simulink model "RoboCup_ARM"  (R2025b)
settings: Solver=FixedStepAuto  StartTime=0.0  StopTime=inf  FixedStep=0.01  RelTol=1e-3
StartFcn:
  | clear attachToRobot
  | clear attachToTool
undefined symbols (not defined in the file or in its folder): gray, q_grip1, Sim3dSensor
libraries: sim3dlib x5, robotsim3dlib x1, robotcorelib x1, robotmaniplib x1, sim3dcameralib x1
settings Model: SimulationMode=accelerator  Creator=Abhishek  LastModifiedBy=FYF
settings DataIOCC: SaveOutput=off  SignalLogging=off  SaveTime=off

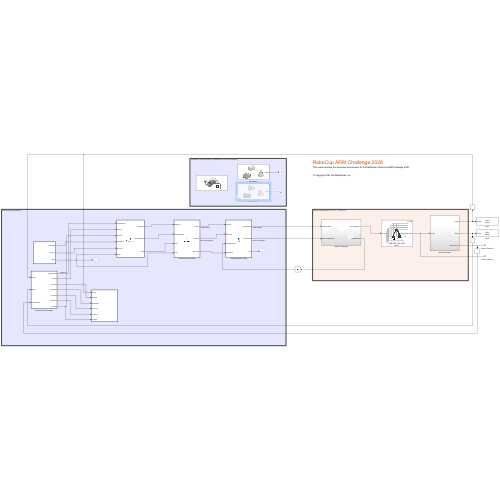
[thumbnail: Simulink's stored preview of the top-level diagram]
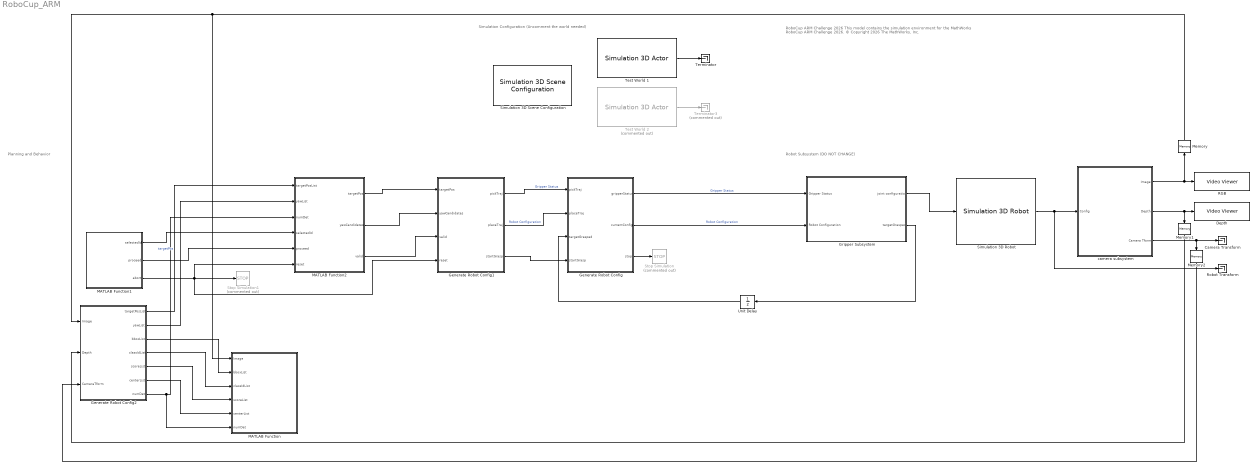
== system RoboCup_ARM ==
  note: Robot Subsystem (DO NOT CHANGE)
  note: Planning and Behavior
  note: Simulation Configuration (Uncomment the world needed)
  note: RoboCup ARM Challenge 2026
      | This model contains the simulation environment for the MathWorks RoboCup ARM Challenge 2026.
      |
      | © Copyright 2026 The MathWorks, Inc.
  Camera Transform : Terminator
  Depth : VideoViewer  colormapValue=gray(256)  FigPos=[1244 879.666666666667 418 304]
  Generate Robot Config : MATLAB Function  TreatAsAtomicUnit=on
  Generate Robot Config1 : MATLAB Function  TreatAsAtomicUnit=on
  Generate Robot Config2 : MATLAB Function  TreatAsAtomicUnit=on
  Gripper Subsystem : Subsystem
  MATLAB Function : MATLAB Function  TreatAsAtomicUnit=on
  MATLAB Function1 : MATLAB Function  TreatAsAtomicUnit=on
  MATLAB Function2 : MATLAB Function  TreatAsAtomicUnit=on
  Memory : Memory
  Memory1 : Memory
  Memory2 : Memory
  "RGB " : VideoViewer  colormapValue=gray(256)  FigPos=[1242 423.666666666667 418 304]
  Robot Transform : Terminator
  Simulation 3D Robot : robotsim3dlib/Simulation 3D Robot  actorInputType=RigidBodyTree Object  RigidBodyTree=rt.robot  ActorName=Robo1  existActorChekBox=on  initialTrans=[0 0 0]  initialRot=[0 0 0]  initialConfig=[-0.2618 -2.1991 1.9722 -1.3963 -1.5882 1.3265 0 0 0 0 0 0]  EndEffector=right_inner_finger_pad  eeOffsetInpChekBox=off  eeTargetTrans=[0 0 0]  eeTargetRot=[0 0 0]  enableRegionGraspChekBox=off  regionGraspInpChekBox=off  eeTargTransDiff=[0.2 0.2 0.2]  eeTargRotDiff=[0 0 0]  enableVisualVisualization=on  enableCollisionVisualization=off  collisionGeomColor=[0 1 0]  collisionGeomTransp=0.1  inpConfEnbVal=on  inpGraspEnbVal=off  inpTransEnbVal=off  outConfEnbVal=on  outGraspEnbVal=off  outTransEnbVal=off  SampleTime=0.01  ActorType=SimulinkVehicle  ID=C  aMode=6  ActorTag=Robo1  Mesh=RigidBodyTree
  Simulation 3D Scene Configuration : sim3dlib/Simulation 3D Scene Configuration  Priority=0  ProjectFormat=Default Scenes  SceneDesc=Empty scene  ProjectName=D:\Program Files\MATLAB\R2025b\toolbox\shared\sim3d_projects\automotive_project_windows\UE\WindowsNoEditor\VehicleSimulation.exe  ScenePath=/Game/Maps/HwStrght  EnableOpenDRIVE=off  vehTagList={'Custom';'Robo1';'Scene Origin';'Sim3dActor1';'Sim3dActor2';'Sim3dActor3';'cameraPlaceHolder'}  vehTag=Scene Origin  AttachedCameraRelativeTranslation=[0 0 0]  FreeCameraDefaultInitialTranslation=[-6, 0, 2]  AttachedCameraRelativeRotation=[0 0 0]  FreeCameraDefaultInitialRotation=[0, -15, 0]  ViewpointName=Custom  FreeCameraInitialTranslation=[0, 0, 0]  ViewpointTranslation=[0 0 0]  FreeCameraInitialRotation=[0, 0, 0]  ViewpointRotation=[0 0 0]  OpVisEn=off  Ts=0.01  EnableWindow=on  EnableRemoteAccess=off  EnableWeather=off  SunAzimuth=90  SunAltitude=40.0  EnableGeospatialSun=off  Latitude=0  Longitude=0  Date=2023-01-01  Time=10:30:00  GeoTimeZone=-5.0  SunDaylightSaving=off  wind=1  clouds=10  EnableVolumetricClouds=off  CloudCoverage=0  CloudAltitude=6  fog=0  rain=0  RaindropsEffect=off  SnowDensity=0  EnableGeospatial=off  TilesetSource=Earth terrain  UseTrueOrigin=off  OriginHeight=200  OriginLatitude=40.744652  OriginLongitude=-73.988864  MapStyle=Aerial  AdditionalAssetIDs=[]  UseAdvancedSunSky=off  SolarTime=11  TimeZone=-5  Day=21  Month=9  Year=2022  UseDaylightSavingTime=on  DSTStartDay=10  DSTStartMonth=3  DSTEndDay=3  DSTEndMonth=11  DSTSwitchHour=2  sensorTag=MainCamera1  sensorId=1  sensorName=MainCamera1  mountLoc=Origin  offsetFlag=off  tmountOffset=[0, 0, 0]  rmountOffset=[0, 0, 0]  HorizontalResolution=1280  VerticalResolution=720  HorizontalFOV=60  mountPoint=[0 0 0]  mountOrientation=[0 0 0]  aMode=5  ID=1  GeoTrigger=Inactive  ViewNameList={'Custom'}  ViewTranslationList={'[0 0 0]'}  ViewRotationList={'[0 0 0]'}
      settings: LibrarySourceBlock=sl3dlib/Simulation 3D/Environment/Simulation 3D Scene Configuration
  Stop Simulation : Stop  Commented=on
  Stop Simulation1 : Stop  Commented=on
  Terminator : Terminator
  Terminator3 : Terminator  Commented=on
  Test World 1 : sim3dlib/Simulation 3D Actor  Priority=1  ActorName=Sim3dActor1  ParentName=Scene Origin  Operation=Create at setup  InitScriptText=|  SampleTime=-1  Translation=[0 0 0]  Rotation=[0 0 0]  Scale=[1 1 1]  aMode=5  ActorTag=Sim3dActor1  ActorType=Sim3dActor  ID=1
      | % Reserved keywords:
      | % - Actor : handle to this actor object
      | % - World : handle to the world object
      | 
      | % Examples:
      | 
      | % Create a primitive geometry (optional)
      | % createShape(Actor, 'box', [1 1 1]);
      | 
      | % Initialize values (optional)
      | % Actor.Physics = true;
      | % Actor.Color = [1 0 0];
      | Actor.load(fullfile(fileparts(get_param(bdroot,'FileName')),'modelData','example_world.mat'))
  Test World 2 : sim3dlib/Simulation 3D Actor  Priority=1  Commented=on  ActorName=Sim3dActor3  ParentName=Scene Origin  Operation=Create at setup  InitScriptText=|  SampleTime=-1  Translation=[0 0 0]  Rotation=[0 0 0]  Scale=[1 1 1]  aMode=5  ActorTag=Sim3dActor3  ActorType=Sim3dActor  ID=3
      | % Reserved keywords:
      | % - Actor : handle to this actor object
      | % - World : handle to the world object
      | 
      | % Examples:
      | 
      | % Create a primitive geometry (optional)
      | % createShape(Actor, 'box', [1 1 1]);
      | 
      | % Initialize values (optional)
      | % Actor.Physics = true;
      | % Actor.Color = [1 0 0];
      | Actor.load(fullfile(fileparts(get_param(bdroot,'FileName')),'modelData','example_world2.mat'))
  Unit Delay : UnitDelay  SampleTime=-1  HasFrameUpgradeWarning=on
  camera subsystem : Subsystem
  wires:
  Gripper Subsystem/1(joint configuration) -> Simulation 3D Robot/1
  Simulation 3D Robot/1 -> Robot Transform/1, camera subsystem/1(Config)
  Generate Robot Config/1(gripperStatus) -> Gripper Subsystem/1(Gripper Status)  "Gripper Status"
  Generate Robot Config/2(currentConfig) -> Gripper Subsystem/2(Robot Configuration)  "Robot Configuration"
  Generate Robot Config/3(stop) -> Stop Simulation/1
  Gripper Subsystem/2(targetGrasped) -> Unit Delay/1
  Unit Delay/1 -> Generate Robot Config/3(targetGrasped)
  Test World 1/1 -> Terminator/1
  camera subsystem/1(Image) -> Memory/1, "RGB "/1
  camera subsystem/2(Depth) -> Memory1/1, Depth/1
  camera subsystem/3(Camera Tform) -> Memory2/1, Camera Transform/1
  Test World 2/1 -> Terminator3/1
  Generate Robot Config2/3(bboxList) -> MATLAB Function/2(bboxList)
  Generate Robot Config2/4(classIdList) -> MATLAB Function/3(classIdList)
  Generate Robot Config2/5(scoreList) -> MATLAB Function/4(scoreList)
  Generate Robot Config2/6(centerList) -> MATLAB Function/5(centerList)
  Generate Robot Config2/7(numDet) -> MATLAB Function/6(numDet), MATLAB Function2/3(numDet)
  Generate Robot Config2/1(targetPosList) -> MATLAB Function2/1(targetPosList)  "targetPos"
  Generate Robot Config2/2(yawList) -> MATLAB Function2/2(yawList)
  MATLAB Function1/1(selectedId) -> MATLAB Function2/4(selectedId)
  MATLAB Function1/2(proceed) -> MATLAB Function2/5(proceed)
  MATLAB Function2/1(targetPos) -> Generate Robot Config1/1(targetPos)
  MATLAB Function2/2(yawCandidates) -> Generate Robot Config1/2(yawCandidates)
  MATLAB Function2/3(valid) -> Generate Robot Config1/3(valid)
  Generate Robot Config1/1(pickTraj) -> Generate Robot Config/1(pickTraj)  "Gripper Status"
  Generate Robot Config1/2(placeTraj) -> Generate Robot Config/2(placeTraj)  "Robot Configuration"
  Memory/1 -> MATLAB Function/1(Image), Generate Robot Config2/1(Image)
  Memory1/1 -> Generate Robot Config2/2(Depth)
  Memory2/1 -> Generate Robot Config2/3(CameraTform)
  MATLAB Function1/3(abort) -> Generate Robot Config1/4(reset), MATLAB Function2/6(reset), Stop Simulation1/1
  Generate Robot Config1/3(startGrasp) -> Generate Robot Config/4(startGrasp)

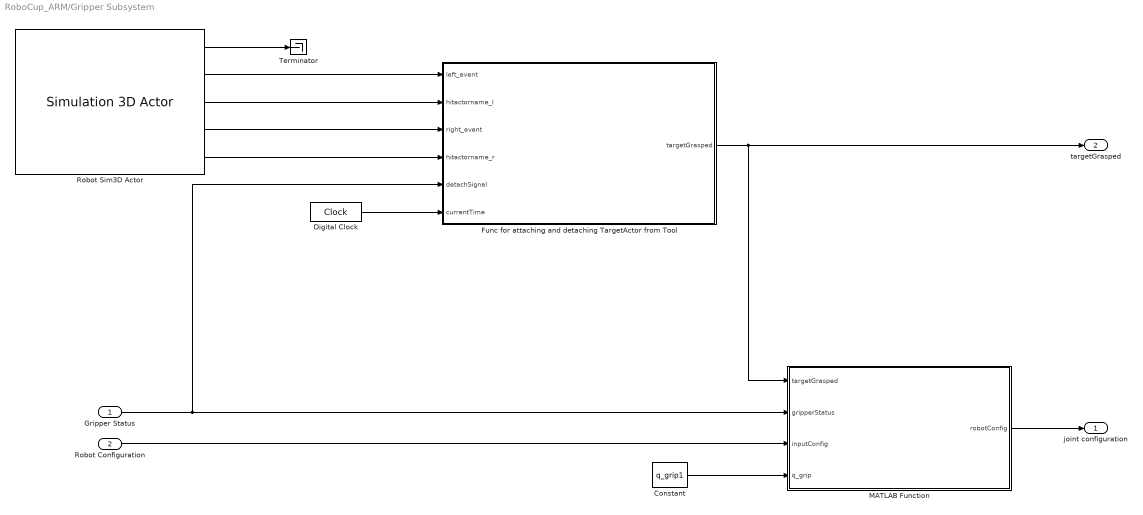
== system RoboCup_ARM/Gripper Subsystem ==
  Gripper Status : Inport
  Robot Configuration : Inport  Port=2
  Constant : Constant  Value=q_grip1
  Digital Clock : DigitalClock
  Func for attaching and detaching TargetActor from Tool : MATLAB Function  TreatAsAtomicUnit=on
  MATLAB Function : MATLAB Function  TreatAsAtomicUnit=on
  Robot Sim3D Actor : sim3dlib/Simulation 3D Actor  Priority=1  ActorName=Sim3dActor2  ParentName=Scene Origin  Operation=Create at setup  InitScriptText=|  SampleTime=-1  Translation=[-0.5 0 1.35]  Rotation=[0 0 0]  Scale=[1 1 1]  EventsText=|  aMode=5  ActorTag=Sim3dActor2  ActorType=Sim3dActor  ID=2
      InitScriptText=|
      | rt = load(fullfile(fileparts(get_param(bdroot,'FileName')),'modelData','ur5e_gripper.mat'));
      | robotActor = sim3d.Actor('ActorName', 'Robo1');
      | World.add(robotActor,Actor);
      | 
      | robotActor.load(rt.robot,[1 1 1]);
      | 
      | % finding tool reference 
      | tool1 = World.Actors.left_inner_finger_pad;
      | tool2 = World.Actors.right_inner_finger_pad;
      | tool1.HitEventEnabled = true;
      | tool1.Collisions = true;
      | 
      | tool2.HitEventEnabled = true;
      | tool2.Collisions = true;
      | 
      | %tool1.Physics = true; % somehow this Phsyics dont work
      | % tool1.Color = [10 0 0];
      | tool1.Mobility =  sim3d.utils.MobilityTypes.Movable;
      | 
      | % tool2.Color = [10 0 0];
      | tool2.Mobility =  sim3d.utils.MobilityTypes.Movable;
      | 
      | propagate(World.Actors.('Sim3dActor2'),'Mobility', sim3d.utils.MobilityTypes.Movable);
      | propagate(World.Actors.('Sim3dActor2'),'Shadows',true);
      EventsText=|
      | left_inner_finger_pad.HitEvent          
      | left_inner_finger_pad.HitOtherActorName 
      | right_inner_finger_pad.HitEvent         
      | right_inner_finger_pad.HitOtherActorName
  Terminator : Terminator
  joint configuration : Outport
  targetGrasped : Outport  Port=2
  wires:
  Robot Sim3D Actor/3 -> Func for attaching and detaching TargetActor from Tool/2(hitactorname_l)
  Robot Sim3D Actor/2 -> Func for attaching and detaching TargetActor from Tool/1(left_event)
  Robot Sim3D Actor/4 -> Func for attaching and detaching TargetActor from Tool/3(right_event)
  Robot Sim3D Actor/5 -> Func for attaching and detaching TargetActor from Tool/4(hitactorname_r)
  Digital Clock/1 -> Func for attaching and detaching TargetActor from Tool/6(currentTime)
  Gripper Status/1 -> Func for attaching and detaching TargetActor from Tool/5(detachSignal), MATLAB Function/2(gripperStatus)
  Robot Configuration/1 -> MATLAB Function/3(inputConfig)
  Func for attaching and detaching TargetActor from Tool/1(targetGrasped) -> MATLAB Function/1(targetGrasped), targetGrasped/1
  Constant/1 -> MATLAB Function/4(q_grip)
  MATLAB Function/1(robotConfig) -> joint configuration/1
  Robot Sim3D Actor/1 -> Terminator/1

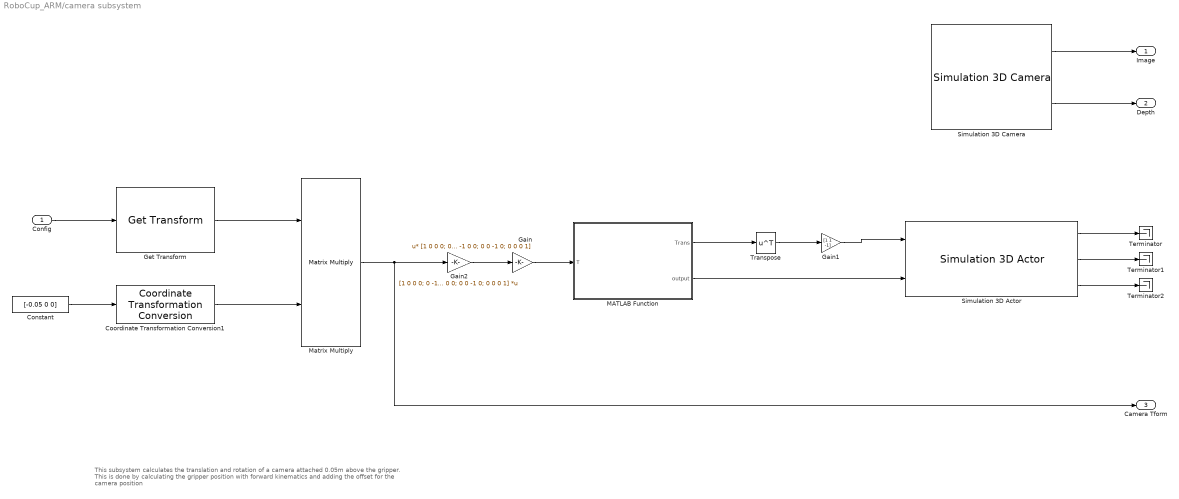
== system RoboCup_ARM/camera subsystem ==
  note: This subsystem calculates the translation and rotation of a camera attached 0.05m above the gripper. This is done by calculating the gripper position with forward kinematics and adding the offset for the camera position
  Config : Inport
  Constant : Constant  Value=[-0.05 0 0]
  Coordinate Transformation Conversion1 : robotcorelib/Coordinate Transformation Conversion  InputRepresentation=Translation Vector  InputEulerSequence=ZYX  ShowTrVecInputPort=on  OutputRepresentation=Homogeneous Transformation  OutputEulerSequence=ZYX  ShowTrVecOutputPort=on  SimulateUsing=Interpreted execution
      settings: LibrarySourceBlock=navlib/Utilities/Coordinate Transformation Conversion
  Gain : Gain  Gain=[1 0 0 0; 0 -1 0 0; 0 0 -1 0; 0 0 0 1]  Multiplication=Matrix(u*K)
  Gain1 : Gain  Gain=[1 1 -1]
  Gain2 : Gain  Gain=[1 0 0 0; 0 -1 0 0; 0 0 -1 0; 0 0 0 1]  Multiplication=Matrix(K*u)
  Get Transform : robotmaniplib/Get Transform  RigidBodyTree=rt.robot  SourceBody=robotiq_arg2f_base_link  TargetBody=base_link  SimulateUsing=Interpreted execution
  MATLAB Function : MATLAB Function  TreatAsAtomicUnit=on
  Matrix Multiply : Product  Multiplication=Matrix(*)
  Simulation 3D Actor : sim3dlib/Simulation 3D Actor  Priority=1  ActorName=cameraPlaceHolder  ParentName=Robo1  Operation=Create at setup  InitScriptText=|  SampleTime=-1  Translation=[0.05 0 0]  Rotation=[0 0 0]  Scale=[1 1 1]  InputsText=cameraPlaceHolder.Translation cameraPlaceHolder.Rotation  OutputsText=cameraPlaceHolder.Translation cameraPlaceHolder.Rotation  aMode=5  ActorTag=cameraPlaceHolder  ActorType=Sim3dActor  ID=C
      | Actor.createShape('box', [0.02 0.04 0.06]);
      | Actor.Mobility=sim3d.utils.MobilityTypes.Movable;
      | Actor.Color=[1 0 0];
      | Actor.Translation=[0.05, 0, 0];
      | Actor.Rotation = [0, 0, 0];
      | Actor.ConstantAttributes=false;
      | Actor.Mass = 1;
      | Actor.Transparency = 0;
      | Actor.Shininess = 0;
  Simulation 3D Camera : sim3dcameralib/Simulation 3D Camera  Priority=1  sensorTag=Sim3dSensor�  sensorId=1  sensorName=Sim3dSensor�  vehTagList={'Robo1';'Scene Origin';'Sim3dActor1';'Sim3dActor2';'Sim3dActor3';'cameraPlaceHolder'}  vehTag=cameraPlaceHolder  CoordinateSystem=ISO8855  mountLoc=Origin  offsetFlag=on  tmountOffset=[0 0 0]  extTmount=off  rmountOffset=[0, -90, 0]  extRmount=off  FocalLength=[1109, 1109]  OpticalCenter=[640, 360]  ImageSize=[720, 1280]  RadialDistortion=[0, 0]  TangentialDistortion=[0, 0]  SensorSkew=0  VisualizeFieldOfView=off  FieldOfViewRange=61  DepthOutportEnabled=on  SemanticOutportEnabled=off  TransformOutportEnabled=off  SampleTime=0.01  mountPoint=[0 0 0]  mountOrientation=[0 -90 0]  aMode=5  ID=1
      settings: LibrarySourceBlock=sl3dlib/Simulation 3D/Sensors/Simulation 3D Camera
  Terminator : Terminator
  Terminator1 : Terminator
  Terminator2 : Terminator
  Transpose : Math  Operator=transpose
  Image : Outport
  Depth : Outport  Port=2
  Camera Tform : Outport  Port=3
  wires:
  MATLAB Function/1(Trans) -> Transpose/1
  Coordinate Transformation Conversion1/1 -> Matrix Multiply/2
  Simulation 3D Actor/2 -> Terminator1/1
  Transpose/1 -> Gain1/1
  Simulation 3D Camera/2 -> Depth/1
  Simulation 3D Actor/1 -> Terminator/1
  Gain/1 -> MATLAB Function/1(T)
  Simulation 3D Actor/3 -> Terminator2/1
  MATLAB Function/2(output) -> Simulation 3D Actor/2
  Matrix Multiply/1 -> Gain2/1, Camera Tform/1
  Gain1/1 -> Simulation 3D Actor/1
  Get Transform/1 -> Matrix Multiply/1
  Simulation 3D Camera/1 -> Image/1
  Gain2/1 -> Gain/1
  Constant/1 -> Coordinate Transformation Conversion1/1
  Config/1 -> Get Transform/1

== matlab function RoboCup_ARM/MATLAB Function2 ==
  data: targetPosList input; targetPos output; yawList input; numDet input; selectedId input; proceed input; yawCandidates output; valid output; reset input
function [targetPos, yawCandidates, valid] = TargetSelect(targetPosList, yawList, numDet, selectedId, proceed, reset)
%#codegen
coder.extrinsic('evalin');
coder.extrinsic('assignin');
coder.extrinsic('fprintf');
coder.extrinsic('cube_target_reset_runtime');
coder.extrinsic('get_cube_place_mode_runtime');

targetPos = zeros(3,1);
yawCandidates = zeros(1,2);
valid = false;

persistent locked latchedTarget latchedYaw lastProceed lastResetToken

if isempty(locked)
    locked = false;
end
if isempty(latchedTarget)
    latchedTarget = zeros(3,1);
end
if isempty(latchedYaw)
    latchedYaw = zeros(1,2);
end
if isempty(lastProceed)
    lastProceed = false;
end
if isempty(lastResetToken)
    lastResetToken = double(0);
end

resetToken = double(0);
resetToken = evalin('base', 'double(USER_RESET_TOKEN)');
tokenReset = (resetToken ~= lastResetToken);

if reset
    locked = false;
    valid = false;
    assignin('base', 'USER_CUBE_ACTIVE', false);
    assignin('base', 'USER_CUBE_SECOND_PICK_PENDING', false);
    assignin('base', 'USER_CUBE_PLACE_MODE', 0);
    assignin('base', 'USER_CUBE_USE_SECOND_HOME', false);
    lastProceed = logical(proceed);
    lastResetToken = resetToken;
    return;
end

if tokenReset
    locked = false;
    valid = false;
    cube_target_reset_runtime();
    lastProceed = logical(proceed);
    lastResetToken = resetToken;
    return;
end


if locked
    targetPos = latchedTarget;
    yawCandidates = latchedYaw;
    valid = true;
    lastProceed = logical(proceed);
    lastResetToken = resetToken;
    return;
end

proceedRise = logical(proceed) && ~logical(lastProceed);
cubePlaceMode = double(0);
cubePlaceMode = get_cube_place_mode_runtime();

if proceedRise && cubePlaceMode == 2
    latchedTarget = [0.799; 0.4; -0.052];
    latchedYaw = [0, 0];

    locked = true;
    assignin('base', 'USER_ACTIVE_TARGET_POS', double(latchedTarget));
    assignin('base', 'USER_ACTIVE_SELECTED_ID', double(1));
    assignin('base', 'USER_CUBE_WAIT_FRESH_VISION', false);
    assignin('base', 'USER_VISION_ENABLE', false);

    targetPos = latchedTarget;
    yawCandidates = latchedYaw;
    valid = true;

    fprintf(['[target_select] SYNTHETIC CUBE SCALE PICK ', ...
        'targetPos=[%.4f %.4f %.4f] yaw=[%.4f %.4f]\n'], ...
        targetPos(1), targetPos(2), targetPos(3), ...
        yawCandidates(1), yawCandidates(2));

elseif proceedRise && selectedId >= 1 && selectedId <= numDet
    latchedTarget = targetPosList(:, selectedId);
    latchedYaw = yawList(:, selectedId).';
    locked = true;

    assignin('base', 'USER_ACTIVE_TARGET_POS', double(latchedTarget));
    assignin('base', 'USER_ACTIVE_SELECTED_ID', double(selectedId));
    assignin('base', 'USER_CUBE_LATCHED_YAW', double(latchedYaw));
    assignin('base', 'USER_VISION_ENABLE', false);

    targetPos = latchedTarget;
    yawCandidates = latchedYaw;
    valid = true;

    fprintf(['[target_select] LATCH selectedId=%d numDet=%d ', ...
        'targetPos=[%.4f %.4f %.4f] yaw=[%.4f %.4f]\n'], ...
        int32(selectedId), int32(numDet), ...
        targetPos(1), targetPos(2), targetPos(3), ...
        yawCandidates(1), yawCandidates(2));
end

lastProceed = logical(proceed);
lastResetToken = resetToken;
end

== matlab function RoboCup_ARM/Gripper Subsystem/MATLAB Function ==
  data: targetGrasped input; robotConfig output; gripperStatus input; inputConfig input; q_grip input
function robotConfig = appendGripper(targetGrasped, gripperStatus, inputConfig, q_grip)

persistent index
if isempty(index)
    index = 1;
end

% Open gripper
if ~gripperStatus
    openConfig = [0 0 0 0 0 0]';
    robotConfig = [inputConfig; openConfig]';
    index = 1;
else
    if index > size(q_grip, 2)
        robotConfig = [inputConfig; q_grip(:, index-1)]';
        index = 1;
    elseif targetGrasped
        robotConfig = [inputConfig; q_grip(:, index)]';
    else
        robotConfig = [inputConfig; q_grip(:, index)]';
        index = index + 1;
    end
end

== matlab function RoboCup_ARM/Gripper Subsystem/Func for attaching and detaching TargetActor from Tool ==
  data: left_event input; targetGrasped output; hitactorname_l input; right_event input; hitactorname_r input; detachSignal input; currentTime input
 function targetGrasped = attachToRobot(left_event, hitactorname_l, right_event, hitactorname_r, detachSignal, currentTime)
    
    persistent l_time r_time grasped;
    if isempty(l_time)
        l_time = 0;
    end

    if isempty(r_time)
        r_time = 1;
    end

    if left_event
        l_time = currentTime;
    end

    if right_event
        r_time = currentTime;
    end
    
    if isempty(grasped)
        grasped = 0;
    end

    targetGrasped = grasped;

    coder.extrinsic('attachToTool');

    if abs(l_time - r_time) < 0.5 || ~detachSignal
        grasped = attachToTool(hitactorname_l, hitactorname_r,detachSignal);
        targetGrasped = grasped;
    end
end

== matlab function RoboCup_ARM/Generate Robot Config ==
  data: pickTraj input size=[6 251]; gripperStatus output size=[1 1]; placeTraj input size=[6 351]; targetGrasped input size=[1 1]; currentConfig output size=[6 1]; stop output size=[1 1]; startGrasp input size=[1 1]
function [gripperStatus, currentConfig, stop] = main(pickTraj, placeTraj, targetGrasped, startGrasp)
%#codegen
coder.extrinsic('assignin');
coder.extrinsic('evalin');
coder.extrinsic('get_cube_place_mode_runtime');
coder.extrinsic('get_user_qhome_current_runtime');
coder.extrinsic('cube_first_drop_runtime');
coder.extrinsic('finish_drop_reset_runtime');
coder.extrinsic('has_pending_view_move_runtime');
coder.extrinsic('finish_view_move_runtime');
coder.extrinsic('get_qhome_next_runtime');
coder.extrinsic('cube_debug_runtime');
coder.extrinsic('record_grasp_failure_runtime');

stop = false;
gripperStatus = 0;

persistent state index delay waitStableCount viewMoveTraj viewMoveIndex viewMoveMode holdConfig holdValid
persistent grabHoldCount

if isempty(state)
    state = 0;
end
if isempty(index)
    index = 1;
end
if isempty(delay)
    delay = 1;
end
if isempty(waitStableCount)
    waitStableCount = uint16(0);
end
if isempty(viewMoveTraj)
    viewMoveTraj = zeros(6,120);
end
if isempty(viewMoveIndex)
    viewMoveIndex = 1;
end
if isempty(viewMoveMode)
    viewMoveMode = 0;
end
if isempty(holdConfig)
    holdConfig = zeros(6,1);
end
if isempty(holdValid)
    holdValid = false;
end
if isempty(grabHoldCount)
    grabHoldCount = uint16(0);
end

DROP_SETTLE_TICKS = 20;
OPEN_SETTLE_TICKS = 30;
RETURN_STEPS = 120;

nPick = size(pickTraj, 2);
nPlace = size(placeTraj, 2);

currentConfig = pickTraj(:,1);

canPick = false;
if state == 0
    if waitStableCount < uint16(65535)
        waitStableCount = waitStableCount + uint16(1);
    end
    canPick = (waitStableCount >= uint16(20));
else
    waitStableCount = uint16(0);
end
assignin('base', 'USER_CAN_PICK', canPick);

if state == 0
    gripperStatus = 0;
    assignin('base', 'USER_VISION_ENABLE', true);
    if holdValid
        currentConfig = holdConfig;
    else
        currentConfig = pickTraj(:,1);
        holdConfig = currentConfig;
        holdValid = true;
    end
    cube_debug_runtime(10, state, canPick, startGrasp, currentConfig);

    hasPendingViewMove = false;
    hasPendingViewMove = has_pending_view_move_runtime();
    qNextView = currentConfig;
    if hasPendingViewMove
        qNextView = get_qhome_next_runtime(currentConfig);
        qStart = currentConfig;
        for k = 1:120
            alpha = (k-1) / (RETURN_STEPS-1);
            viewMoveTraj(:,k) = (1-alpha)*qStart + alpha*qNextView;
        end
        viewMoveIndex = 1;
        viewMoveMode = 1;
        holdValid = false;
        state = 6;
        waitStableCount = uint16(0);
        assignin('base', 'USER_VISION_ENABLE', false);
        return;
    end

    if startGrasp
        cube_debug_runtime(30, state, canPick, startGrasp, currentConfig);
        assignin('base', 'USER_VISION_ENABLE', false);
        state = 1;
        index = 1;
        delay = 1;
        waitStableCount = uint16(0);
        holdValid = false;
        grabHoldCount = uint16(0);
    end
    return;
end

if state == 1
    gripperStatus = 0;
    assignin('base', 'USER_VISION_ENABLE', false);
    currentConfig = pickTraj(:, index);
    holdConfig = currentConfig;
    holdValid = true;
    index = index + 1;
    if index > nPick
        state = 2;
        index = nPick;
        grabHoldCount = uint16(0);
    end

elseif state == 2
    gripperStatus = 1;
    assignin('base', 'USER_VISION_ENABLE', false);
    currentConfig = pickTraj(:, index);
    holdConfig = currentConfig;
    holdValid = true;
    if grabHoldCount < uint16(65535)
        grabHoldCount = grabHoldCount + uint16(1);
    end

    if targetGrasped
        state = 3;
        index = 1;
        grabHoldCount = uint16(0);
    else
        grabTimeoutFrames = uint16(180);
        tmpExist = double(0);
        tmpExist = evalin('base', 'double(exist(''USER_GRAB_TIMEOUT_FRAMES'',''var''))');
        if tmpExist ~= 0
            t = double(180);
            t = evalin('base', 'double(USER_GRAB_TIMEOUT_FRAMES)');
            if isfinite(t) && t >= 10
                if t > 1000
                    t = 1000;
                end
                grabTimeoutFrames = uint16(round(t));
            end
        end

        if grabHoldCount >= grabTimeoutFrames
            record_grasp_failure_runtime();

            qStart = currentConfig;
            qHomeNow = pickTraj(:,1);
            for k = 1:120
                alpha = (k-1) / (RETURN_STEPS-1);
                viewMoveTraj(:,k) = (1-alpha)*qStart + alpha*qHomeNow;
            end
            viewMoveIndex = 1;
            viewMoveMode = 0;
            holdValid = false;
            gripperStatus = 0;
            state = 6;
            index = 1;
            delay = 1;
            waitStableCount = uint16(0);
            grabHoldCount = uint16(0);
            return;
        end
    end

elseif state == 3
    gripperStatus = 1;
    assignin('base', 'USER_VISION_ENABLE', false);
    currentConfig = placeTraj(:, index);
    holdConfig = currentConfig;
    holdValid = true;
    index = index + 1;
    if index > nPlace
        state = 7;
        index = nPlace;
        delay = 1;
    end

elseif state == 7
    gripperStatus = 1;
    assignin('base', 'USER_VISION_ENABLE', false);
    currentConfig = placeTraj(:, index);
    holdConfig = currentConfig;
    holdValid = true;
    if delay <= DROP_SETTLE_TICKS
        delay = delay + 1;
    else
        state = 4;
    end

elseif state == 4
    gripperStatus = 0;
    assignin('base', 'USER_VISION_ENABLE', false);
    currentConfig = placeTraj(:, index);
    holdConfig = currentConfig;
    holdValid = true;
    state = 5;
    delay = 1;

elseif state == 5
    gripperStatus = 0;
    assignin('base', 'USER_VISION_ENABLE', false);
    currentConfig = placeTraj(:, index);
    holdConfig = currentConfig;
    holdValid = true;

    if delay <= OPEN_SETTLE_TICKS
        delay = delay + 1;
        return;
    end

    cubePlaceMode = 0;
    cubePlaceMode = get_cube_place_mode_runtime();

    if cubePlaceMode == 1
        cube_first_drop_runtime(currentConfig);
        cube_debug_runtime(20, state, canPick, startGrasp, currentConfig);
        holdConfig = currentConfig;
        holdValid = true;
        state = 0;
        index = 1;
        delay = 1;
        waitStableCount = uint16(0);
        return;
    end

    qHomeNow = pickTraj(:,1);
    if cubePlaceMode == 2
        qHomeNow = get_user_qhome_current_runtime(qHomeNow);
    end

    qStart = currentConfig;
    for k = 1:120
        alpha = (k-1) / (RETURN_STEPS-1);
        viewMoveTraj(:,k) = (1-alpha)*qStart + alpha*qHomeNow;
    end
    viewMoveIndex = 1;
    viewMoveMode = 0;
    holdValid = false;
    state = 6;
    index = 1;
    delay = 1;
    waitStableCount = uint16(0);

elseif state == 6
    gripperStatus = 0;
    assignin('base', 'USER_VISION_ENABLE', false);
    currentConfig = viewMoveTraj(:, viewMoveIndex);
    holdConfig = currentConfig;
    holdValid = true;
    viewMoveIndex = viewMoveIndex + 1;
    if viewMoveIndex > 120
        currentConfig = viewMoveTraj(:,120);
        holdConfig = currentConfig;
        holdValid = true;
        if viewMoveMode == 1
            finish_view_move_runtime(currentConfig);
        else
            finish_drop_reset_runtime();
            assignin('base', 'USER_VISION_ENABLE', true);
        end
        cube_debug_runtime(40, state, canPick, startGrasp, currentConfig);
        state = 0;
        viewMoveIndex = 1;
        viewMoveMode = 0;
        waitStableCount = uint16(0);
    end
end
end

== matlab function RoboCup_ARM/Generate Robot Config1 ==
  data: targetPos input; yawCandidates input; pickTraj output; valid input; placeTraj output; startGrasp output; reset input
function [pickTraj, placeTraj, startGrasp] = planner(targetPos, yawCandidates, valid, reset)
%#codegen

coder.extrinsic('planner_core');
coder.extrinsic('evalin');
coder.extrinsic('fprintf');

pickTraj   = zeros(6,251);
placeTraj  = zeros(6,351);
startGrasp = false;

persistent lastValid planned latchedPick latchedPlace lastResetToken

if isempty(lastValid)
    lastValid = false;
end
if isempty(planned)
    planned = false;
end
if isempty(latchedPick)
    latchedPick = zeros(6,251);
end
if isempty(latchedPlace)
    latchedPlace = zeros(6,351);
end
if isempty(lastResetToken)
    lastResetToken = double(0);
end

resetToken = double(0);
resetToken = evalin('base', 'double(USER_RESET_TOKEN)');
tokenReset = (resetToken ~= lastResetToken);

% reset from manual abort or from auto-loop token
if reset || tokenReset
    planned = false;
    lastValid = false;
    latchedPick  = zeros(6,251);
    latchedPlace = zeros(6,351);
    lastResetToken = resetToken;

    dbgprintf('[planner] reset -> clear latched trajectories\n');
    return;
end

% one pulse when target becomes valid
startGrasp = logical(valid) && ~logical(lastValid);

% plan once then latch
if startGrasp && ~planned
    fprintf(['[planner_start] startGrasp=1 targetPos=[%.4f %.4f %.4f] ', ...
        'yaw=[%.4f %.4f]\n'], ...
        targetPos(1), targetPos(2), targetPos(3), ...
        yawCandidates(1), yawCandidates(2));
    [latchedPick, latchedPlace] = planner_core(targetPos, yawCandidates, true);
    planned = true;
    dbgprintf('[planner] trajectory planned and latched once.\n');
end

if planned
    pickTraj  = latchedPick;
    placeTraj = latchedPlace;
else
    [pickTraj, placeTraj] = planner_core(targetPos, yawCandidates, false);
end

dbgprintf('[planner] valid=%.0f lastValid=%.0f startGrasp=%.0f planned=%.0f\n', ...
    double(valid), double(lastValid), double(startGrasp), double(planned));

lastValid = logical(valid);
lastResetToken = resetToken;

end

function dbgprintf(varargin)
% suppress per-step console output
end

== matlab function RoboCup_ARM/camera subsystem/MATLAB Function ==
  data: T input; Trans output; output output
function [Trans, output] = rotm2fixedZYX(T)
    R = T(1:3,1:3);
    Trans = T(1:3,4);
    if abs(R(3,1)) < 1
        pitch = -asin(R(3,1));
        roll  = atan2(R(3,2)/cos(pitch), R(3,3)/cos(pitch));
        yaw   = atan2(R(2,1)/cos(pitch), R(1,1)/cos(pitch));
    else
        % Gimbal lock
        if R(3,1) <= -1
            pitch = pi/2;
        else
            pitch = -pi/2;
        end
        yaw = 0;
        roll = atan2(-R(1,2), R(1,3));
    end
    output = [roll, pitch, yaw];
end

== matlab function RoboCup_ARM/Generate Robot Config2 ==
  data: Image input; targetPosList output; yawList output; Depth input; CameraTform input; bboxList output; classIdList output; scoreList output; centerList output; numDet output
function [targetPosList, yawList, bboxList, classIdList, scoreList, centerList, numDet] = ...
    vision(Image, Depth, CameraTform)
%#codegen
coder.extrinsic('vision_core_multi');
coder.extrinsic('assignin');

targetPosList = zeros(3,20);
yawList       = zeros(2,20);
bboxList      = zeros(4,20);
classIdList   = zeros(1,20);
scoreList     = zeros(1,20);
centerList    = zeros(2,20);
numDet        = 0;

[targetPosList, yawList, bboxList, classIdList, scoreList, centerList, numDet] = ...
    vision_core_multi(Image, Depth, CameraTform);

% Publish latest detection count for UserCommand auto-loop gate.
assignin('base', 'VISION_LAST_NUMDET', double(numDet));
end

== matlab function RoboCup_ARM/MATLAB Function ==
  data: Image input; bboxList input; classIdList input; scoreList input; centerList input; numDet input
function preview_block(Image, bboxList, classIdList, scoreList, centerList, numDet)
%#codegen
coder.extrinsic('vision_preview');

MAXDET = 20;
yawList = zeros(2, MAXDET);
for i = 1:MAXDET
    yawList(:,i) = [0; pi/2];
end

vision_preview(Image, bboxList, classIdList, scoreList, centerList, yawList, numDet);
end

== matlab function RoboCup_ARM/MATLAB Function1 ==
  data: selectedId output; proceed output; abort output
function [selectedId, proceed, abort] = UserCommand()
%#codegen
coder.extrinsic('user_command_runtime');

selectedId = double(0);
proceed = false;
abort = false;

sid = double(0);
pr = false;
ab = false;

[sid, pr, ab] = user_command_runtime();

selectedId = double(sid);
proceed = logical(pr);
abort = logical(ab);
end
